simulink model "modelagem"  (R2020a)
settings: Solver=FixedStepDiscrete  StartTime=0.0  StopTime=inf  FixedStep=0.01  RelTol=1e-3
values from neighbouring files (symbols this model uses):
  ISA_AND = uint8(48)    [load_constants.m]
  ISA_B_PUSH = uint8(64)    [load_constants.m]
  ISA_CTD = uint8(97)    [load_constants.m]
  ISA_CTU = uint8(96)    [load_constants.m]
  ISA_END = uint8(0)    [load_constants.m]
  ISA_JMP = uint8(112)    [load_constants.m]
  ISA_LD = uint8(16)    [load_constants.m]
  ISA_LDN = uint8(17)    [load_constants.m]
  ISA_NOT = uint8(50)    [load_constants.m]
  ISA_OR = uint8(49)    [load_constants.m]
  ISA_OUT = uint8(32)    [load_constants.m]
  ISA_RST = uint8(34)    [load_constants.m]
  ISA_RSTC = uint8(98)    [load_constants.m]
  ISA_SET = uint8(33)    [load_constants.m]
  ISA_TOF = uint8(81)    [load_constants.m]
  ISA_TON = uint8(80)    [load_constants.m]
  ISA_TP = uint8(82)    [load_constants.m]
  Program = zeros(1, MEM_PROG_SIZE, 'uint8')    [setup_clp.m]
  TIM_PRES_LIM = 4000000000    [load_constants.m]
settings Model: EnablePacing=on  Creator=gabri  LastModifiedBy=gabri

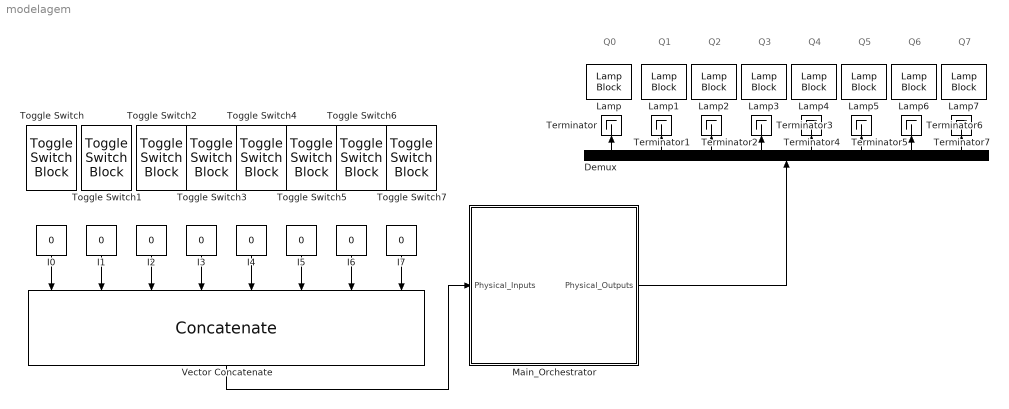
== system modelagem ==
  note: Q0
  note: Q1
  note: Q2
  note: Q3
  note: Q4
  note: Q5
  note: Q6
  note: Q7
  Demux : Demux  Outputs=8
  I{0..7} (8 alike) : Constant  Value=0  OutDataTypeStr=uint8
  Lamp{,1..7} (8 alike) : LampBlock
  Main_Orchestrator : Stateflow chart  TreatAsAtomicUnit=on
  Terminator{,1..7} (8 alike) : Terminator
  Toggle Switch{,1..7} (8 alike) : ToggleSwitchBlock
      settings: Values={{'Off', 'On'}, [0 1]}
  Vector Concatenate : Concatenate  NumInputs=8
  wires:
  I0/1 -> Vector Concatenate/1
  I1/1 -> Vector Concatenate/2
  I2/1 -> Vector Concatenate/3
  I3/1 -> Vector Concatenate/4
  I4/1 -> Vector Concatenate/5
  I5/1 -> Vector Concatenate/6
  I6/1 -> Vector Concatenate/7
  I7/1 -> Vector Concatenate/8
  Vector Concatenate/1 -> Main_Orchestrator/1(Physical_Inputs)
  Demux/1 -> Terminator/1
  Demux/2 -> Terminator1/1
  Demux/3 -> Terminator2/1
  Demux/4 -> Terminator3/1
  Demux/5 -> Terminator4/1
  Demux/6 -> Terminator5/1
  Demux/7 -> Terminator6/1
  Demux/8 -> Terminator7/1
  Main_Orchestrator/1(Physical_Outputs) -> Demux/1

== stateflow chart modelagem/Main_Orchestrator ==
  settings: updateMethod=DISCRETE  sampleTime=0.01
  state READ_INPUTS
    entry:
    Input_Image = Physical_Inputs;
  state EXECUTE_VM
    state INIT_VM
      entry:
      Scan_Complete = 0;
      Stack_Pointer = -1;
      Instruction_Pointer = 0;
    state EXECUTION_HUB
      entry:
      state UNIT_IO
        state EXEC_LD
          entry:
          Instruction_Pointer++;
          Stack_Pointer = 0;
          addr = Program[Instruction_Pointer];
          Instruction_Pointer++;
        state EXEC_LDN
          entry:
          Instruction_Pointer++;
          Stack_Pointer = 0;
          addr = Program[Instruction_Pointer];
          Instruction_Pointer++;
        state EXEC_OUT
          entry:
          Instruction_Pointer++;
          Output_Image[ Program[Instruction_Pointer] ] = Stack[Stack_Pointer];
          Instruction_Pointer++;
        state EXEC_SET
          entry:
          Instruction_Pointer++;
        state EXEC_RST
          entry:
          Instruction_Pointer++;
        state END_OF_LINE
          entry:
          Hub_Complete = 1;
        EXEC_LD -> (junction 487)
        (junction 487) -> (junction 490) [order 2] : {Stack[Stack_Pointer] = Input_Image[addr];}
        (junction 487) -> (junction 489) [order 1] : [addr >= 128]
        (junction 490) -> (junction 320)
        (default) -> (junction 223)
        (junction 223) -> EXEC_LD [order 1] : [Current_Inst == ISA_LD]
        (junction 223) -> (junction 229) [order 2]
        (junction 489) -> (junction 320) : {Stack[Stack_Pointer] = Output_Image[addr - 128];}
        (junction 320) -> (junction 500)
        (junction 502) -> (junction 500) [order 2] : {Stack[Stack_Pointer] = !Input_Image[addr];}
        EXEC_LDN -> (junction 502)
        (junction 502) -> (junction 496) [order 1] : [addr >= 128]
        (junction 500) -> (junction 498)
        (junction 229) -> EXEC_LDN [order 1] : [Current_Inst == ISA_LDN]
        (junction 229) -> (junction 233) [order 2]
        (junction 496) -> (junction 498) : {Stack[Stack_Pointer] = !Output_Image[addr - 128];}
        (junction 498) -> (junction 322)
        (junction 233) -> EXEC_OUT [order 1] : [Current_Inst == ISA_OUT]
        EXEC_OUT -> (junction 322)
        (junction 233) -> (junction 347) [order 2]
        (junction 322) -> (junction 362)
        (junction 358) -> (junction 361) : {Output_Image[ Program[Instruction_Pointer] ] = 1;}
        (junction 355) -> (junction 358) [order 1] : [Stack[Stack_Pointer] == 1]
        (junction 361) -> (junction 323)
        EXEC_SET -> (junction 355)
        (junction 355) -> (junction 323) [order 2]
        (junction 323) -> (junction 362) : {Instruction_Pointer++;}
        (junction 347) -> EXEC_SET [order 1] : [Current_Inst == ISA_SET]
        (junction 362) -> (junction 380)
        (junction 347) -> (junction 352) [order 2]
        (junction 377) -> (junction 370) : {Output_Image[ Program[Instruction_Pointer] ] = 0;}
        (junction 376) -> (junction 377) [order 1] : [Stack[Stack_Pointer] == 1]
        (junction 370) -> (junction 378)
        EXEC_RST -> (junction 376)
        (junction 376) -> (junction 378) [order 2]
        (junction 378) -> (junction 380) : {Instruction_Pointer++;}
        (junction 352) -> EXEC_RST [order 1] : [Current_Inst == ISA_RST]
        (junction 380) -> (junction 383)
        (junction 352) -> EXECUTE_VM.EXECUTION_HUB.UNIT_IO.END_OF_LINE [order 2]
        (junction 383) -> EXECUTE_VM.EXECUTION_HUB.UNIT_IO.END_OF_LINE
      state UNIT_LOGIC
        state EXEC_AND
          entry:
          Instruction_Pointer++;
          Stack[Stack_Pointer] = Stack[Stack_Pointer] && Input_Image[ Program[Instruction_Pointer] ];
          Instruction_Pointer++;
        state EXEC_OR
          entry:
          Instruction_Pointer++;
          Stack[Stack_Pointer] = Stack[Stack_Pointer] || Input_Image[ Program[Instruction_Pointer] ];
          Instruction_Pointer++;
        state EXEC_NOT
          entry:
          Stack[Stack_Pointer] = !Stack[Stack_Pointer];
          Instruction_Pointer++;
        state END_OF_LINE
          entry:
          Hub_Complete = 1;
        (default) -> (junction 248)
        (junction 248) -> EXEC_AND [order 1] : [Current_Inst == ISA_AND]
        EXEC_AND -> (junction 331)
        (junction 248) -> (junction 239) [order 2]
        (junction 331) -> (junction 332)
        (junction 239) -> EXEC_OR [order 1] : [Current_Inst == ISA_OR]
        EXEC_OR -> (junction 332)
        (junction 239) -> (junction 243) [order 2]
        (junction 332) -> (junction 333)
        (junction 243) -> EXEC_NOT [order 1] : [Current_Inst == ISA_NOT]
        EXEC_NOT -> (junction 333)
        (junction 243) -> EXECUTE_VM.EXECUTION_HUB.UNIT_LOGIC.END_OF_LINE [order 2]
        (junction 333) -> (junction 335)
        (junction 335) -> EXECUTE_VM.EXECUTION_HUB.UNIT_LOGIC.END_OF_LINE
      state UNIT_STACK
      state UNIT_TIMERS
        state EXEC_TON
          entry:
          Instruction_Pointer++;
          t_idx = Program[Instruction_Pointer];
          Instruction_Pointer++;
          t_pre = Program[Instruction_Pointer];
          Instruction_Pointer++;
        state EXEC_TOF
          entry:
          Instruction_Pointer++;
          t_idx = Program[Instruction_Pointer];
          Instruction_Pointer++;
          t_pre = Program[Instruction_Pointer];
          Instruction_Pointer++;
        state EXEC_TP
          entry:
          Instruction_Pointer++;
          t_idx = Program[Instruction_Pointer];
          Instruction_Pointer++;
          t_pre = Program[Instruction_Pointer];
          Instruction_Pointer++;
          t_val = Stack[Stack_Pointer];
        state END_OF_LINE
          entry:
          Hub_Complete = 1;
        EXEC_TON -> (junction 294)
        (junction 293) -> (junction 299) [order 1] : [Timer_Acc[t_idx] >= TIM_PRES_LIM]
        (junction 294) -> (junction 293) [order 1] : [Stack[Stack_Pointer] == 1]
        (junction 299) -> (junction 297)
        (junction 294) -> (junction 298) [order 2] : {Timer_Acc[t_idx] = 0;}
        (junction 293) -> (junction 289) [order 2] : {Timer_Acc[t_idx] = Timer_Acc[t_idx] + 1;}
        (default) -> (junction 282)
        (junction 282) -> EXEC_TON [order 1] : [Current_Inst == ISA_TON]
        (junction 282) -> (junction 421) [order 2]
        (junction 297) -> (junction 289)
        (junction 289) -> (junction 298)
        (junction 298) -> (junction 290)
        (junction 290) -> (junction 296) [order 1] : [Timer_Acc[t_idx] >= t_pre]
        (junction 290) -> (junction 300) [order 2] : {Stack[Stack_Pointer] = 0;}
        (junction 296) -> (junction 292) : {Stack[Stack_Pointer] = 1;}
        (junction 300) -> (junction 292)
        (junction 292) -> (junction 343)
        (junction 343) -> (junction 417)
        EXEC_TOF -> (junction 397)
        (junction 397) -> (junction 399) [order 1] : [Stack[Stack_Pointer] == 1]
        (junction 399) -> (junction 403) : {Timer_Acc[t_idx] = t_pre;
            | Stack[Stack_Pointer] = 1;}
        (junction 397) -> (junction 400) [order 2]
        (junction 403) -> (junction 411)
        (junction 421) -> EXEC_TOF [order 1] : [Current_Inst == ISA_TOF]
        (junction 400) -> (junction 405) [order 1] : [Timer_Acc[t_idx] > 0]
        (junction 405) -> (junction 411) : {Timer_Acc[t_idx]--;
            | Stack[Stack_Pointer] = 1;}
        (junction 411) -> (junction 417)
        (junction 421) -> (junction 426) [order 2]
        (junction 400) -> (junction 407) [order 2]
        (junction 413) -> (junction 411)
        (junction 417) -> (junction 481)
        (junction 407) -> (junction 409) : {Stack[Stack_Pointer] = 0;}
        (junction 409) -> (junction 413)
        (junction 471) -> (junction 473) : {Timer_Acc[t_idx] = 0;}
        (junction 469) -> (junction 471) [order 1] : [Stack[Stack_Pointer] == 0]
        (junction 473) -> (junction 476)
        EXEC_TP -> (junction 442)
        (junction 442) -> (junction 453) [order 1] : [t_val == 1 && Timer_Acc[t_idx] == 0]
        (junction 461) -> (junction 469) : {Stack[Stack_Pointer] = 0;}
        (junction 469) -> (junction 476) [order 2]
        (junction 442) -> (junction 449) [order 2]
        (junction 453) -> (junction 438) : {Timer_Acc[t_idx] = 1;}
        (junction 456) -> (junction 461) [order 2]
        (junction 476) -> (junction 465)
        (junction 426) -> EXEC_TP [order 1] : [Current_Inst == ISA_TP]
        (junction 426) -> EXECUTE_VM.EXECUTION_HUB.UNIT_TIMERS.END_OF_LINE [order 2]
        (junction 449) -> (junction 438)
        (junction 438) -> (junction 456) [order 1] : [Timer_Acc[t_idx] > 0]
        (junction 456) -> (junction 462) [order 1] : [Timer_Acc[t_idx] < t_pre]
        (junction 462) -> (junction 465) : {Timer_Acc[t_idx] = Timer_Acc[t_idx] + 1;
            |         Stack[Stack_Pointer] = 1;}
        (junction 465) -> (junction 481)
        (junction 438) -> (junction 459) [order 2] : {Stack[Stack_Pointer] = 0;}
        (junction 467) -> (junction 465)
        (junction 481) -> (junction 393)
        (junction 459) -> (junction 467)
        (junction 393) -> EXECUTE_VM.EXECUTION_HUB.UNIT_TIMERS.END_OF_LINE
      state UNIT_COUNTERS
        state EXEC_CTU
          entry:
          Instruction_Pointer++; c_idx = Program[Instruction_Pointer];
          Instruction_Pointer++; c_pre = Program[Instruction_Pointer];
          Instruction_Pointer++;
          input_val = Stack[Stack_Pointer];
        state EXEC_CTD
          entry:
          Instruction_Pointer++; c_idx = Program[Instruction_Pointer];
          Instruction_Pointer++; c_pre = Program[Instruction_Pointer];
          Instruction_Pointer++;
          input_val = Stack[Stack_Pointer];
        state EXEC_RSTC
          entry:
          Instruction_Pointer++; c_idx = Program[Instruction_Pointer];
          Instruction_Pointer++;
        state END_OF_LINE
          entry:
          Hub_Complete = 1;
        (junction 622) -> (junction 674) : {Stack[Stack_Pointer] = 1;}
        (junction 617) -> (junction 622) [order 1] : [Counter_Acc[c_idx] >= c_pre]
        (junction 674) -> (junction 619)
        (default) -> (junction 519)
        (junction 617) -> (junction 619) [order 2] : {Stack[Stack_Pointer] = 0;}
        EXEC_CTU -> (junction 518)
        (junction 518) -> (junction 617) [order 2]
        (junction 619) -> (junction 624) : {Counter_Prev_Up[c_idx] = input_val;}
        (junction 518) -> (junction 610) [order 1] : [input_val == 1 && Counter_Prev_Up[c_idx] == 0]
        (junction 614) -> (junction 617)
        (junction 624) -> (junction 643)
        (junction 519) -> EXEC_CTU [order 1] : [Current_Inst == ISA_CTU]
        (junction 519) -> (junction 543) [order 2]
        (junction 610) -> (junction 614) : {Counter_Acc[c_idx] = Counter_Acc[c_idx] + 1;}
        (junction 630) -> (junction 676) : {Stack[Stack_Pointer] = 1;}
        (junction 635) -> (junction 630) [order 1] : [Counter_Acc[c_idx] <= 0]
        (junction 676) -> (junction 677)
        EXEC_CTD -> (junction 636)
        (junction 636) -> (junction 635) [order 2]
        (junction 635) -> (junction 677) [order 2] : {Stack[Stack_Pointer] = 0;}
        (junction 677) -> (junction 643) : {Counter_Prev_Down[c_idx] = input_val;}
        (junction 636) -> (junction 648) [order 1] : [input_val == 1 && Counter_Prev_Down[c_idx] == 0]
        (junction 632) -> (junction 635)
        (junction 643) -> (junction 644)
        (junction 543) -> EXEC_CTD [order 1] : [Current_Inst == ISA_CTD]
        (junction 543) -> (junction 555) [order 2]
        (junction 648) -> (junction 632) [order 2]
        (junction 648) -> (junction 650) [order 1] : [Counter_Acc[c_idx] > 0]
        (junction 631) -> (junction 632)
        (junction 644) -> (junction 668)
        (junction 650) -> (junction 631) : {Counter_Acc[c_idx] = Counter_Acc[c_idx] - 1;}
        EXEC_RSTC -> (junction 657)
        (junction 657) -> (junction 661) [order 2]
        (junction 661) -> (junction 668)
        (junction 657) -> (junction 659) [order 1] : [Stack[Stack_Pointer] == 1]
        (junction 663) -> (junction 661)
        (junction 668) -> (junction 553)
        (junction 555) -> EXEC_RSTC [order 1] : [Current_Inst == ISA_RSTC]
        (junction 555) -> EXECUTE_VM.EXECUTION_HUB.UNIT_COUNTERS.END_OF_LINE [order 2]
        (junction 659) -> (junction 664) : {Counter_Acc[c_idx] = 0;}
        (junction 664) -> (junction 663) : {Counter_Prev_Up[c_idx] = 0;
            | Counter_Prev_Down[c_idx] = 0;}
        (junction 553) -> EXECUTE_VM.EXECUTION_HUB.UNIT_COUNTERS.END_OF_LINE
      state UNIT_FLOW
      state EXEC_NOP
        entry:
        Hub_Complete = 1;
      state HUB_DONE
      (default) -> (junction 174)
      (junction 174) -> UNIT_IO [order 1] : [Current_Inst >= ISA_LD && Current_Inst < ISA_AND]
      UNIT_IO -> (junction 205)
      (junction 174) -> (junction 178) [order 2]
      (junction 205) -> (junction 206)
      UNIT_LOGIC -> (junction 206)
      (junction 178) -> UNIT_LOGIC [order 1] : [Current_Inst >= ISA_AND && Current_Inst < ISA_B_PUSH]
      (junction 206) -> (junction 207)
      (junction 178) -> (junction 182) [order 2]
      (junction 182) -> UNIT_STACK [order 1] : [Current_Inst >= ISA_B_PUSH && Current_Inst < ISA_TON]
      UNIT_STACK -> (junction 207)
      (junction 182) -> (junction 187) [order 2]
      (junction 207) -> (junction 208)
      (junction 187) -> UNIT_TIMERS [order 1] : [Current_Inst >= ISA_TON && Current_Inst < ISA_CTU]
      UNIT_TIMERS -> (junction 208)
      (junction 187) -> (junction 191) [order 2]
      (junction 208) -> (junction 209)
      (junction 191) -> UNIT_COUNTERS [order 1] : [Current_Inst >= ISA_CTU && Current_Inst < ISA_JMP]
      UNIT_COUNTERS -> (junction 209)
      (junction 191) -> (junction 195) [order 2]
      (junction 209) -> (junction 210)
      UNIT_FLOW -> (junction 210)
      (junction 195) -> UNIT_FLOW [order 1] : [Current_Inst >= ISA_JMP]
      (junction 210) -> (junction 316)
      (junction 195) -> EXEC_NOP [order 2]
      EXEC_NOP -> (junction 316)
      (junction 316) -> HUB_DONE : [Hub_Complete == 1]
    state FETCH
      entry:
      Current_Inst = Program[Instruction_Pointer];
      Hub_Complete = 0;
    state VM_DONE
      entry:
      Scan_Complete = 1;
    EXECUTION_HUB -> FETCH : [Hub_Complete == 1]
    (default) -> INIT_VM
    FETCH -> EXECUTION_HUB [order 1] : [Current_Inst != ISA_END]
    INIT_VM -> FETCH
    FETCH -> (junction 171) [order 2] : [Current_Inst == ISA_END]
    (junction 171) -> VM_DONE
  state WRITE_OUTPUTS
    entry:
    Physical_Outputs = Output_Image;
  (default) -> READ_INPUTS
  WRITE_OUTPUTS -> READ_INPUTS
  READ_INPUTS -> EXECUTE_VM
  EXECUTE_VM -> WRITE_OUTPUTS : [Scan_Complete == 1]
  data: Physical_Inputs input uint8 size=[8]; Physical_Outputs output uint8 size=[8]; Input_Image local uint8 size=[8]; Stack local boolean size=[8]; Stack_Pointer local int8 size=1; Instruction_Pointer local uint8 size=1; Program parameter uint8 size=[64]; Current_Inst local uint8 size=1; Scan_Complete local uint8 size=1; ISA_LD parameter; ISA_AND parameter; ISA_END parameter; ISA_OR parameter; ISA_OUT parameter; ISA_LDN parameter; ISA_NOT parameter; Output_Image local uint8 size=[8]; Timer_Acc local uint32 size=[8] =zeros(1,8); t_idx local uint8 size=1; t_pre local uint32 size=1; ISA_TON parameter; TIM_PRES_LIM parameter; Hub_Complete local uint8; ISA_B_PUSH parameter; ISA_CTU parameter; ISA_JMP parameter; ISA_RST parameter; ISA_SET parameter; t_val local uint8; ISA_TOF parameter; ISA_TP parameter; addr local uint8; Counter_Acc local uint32 size=[8]; Counter_Prev_Up local uint8 size=[8]; input_val local uint8; c_idx local uint8; c_pre local uint32; ISA_CTD parameter; ISA_RSTC parameter; Counter_Prev_Down local uint8 size=[8]
